simulink model "HighLevelControl2"  (R2020a)
settings: Solver=FixedStepAuto  StartTime=0.0  StopTime=10  FixedStep=0.01  RelTol=1e-3
libraries: fuzblock x1
settings Model: Creator=Sarah Bassem  LastModifiedBy=ElMousel
settings SolverCC: ZeroCrossControl=DisableAll
settings DataIOCC: ReturnWorkspaceOutputs=off
settings DebuggingCC: ArithmeticOperatorsInVariantConditions=warning
settings SFSimCC: SimUseLocalCustomCode=off  CustomCodeUndefinedFunction=UseInterfaceOnly
settings RTWCC: RTWUseLocalCustomCode=off

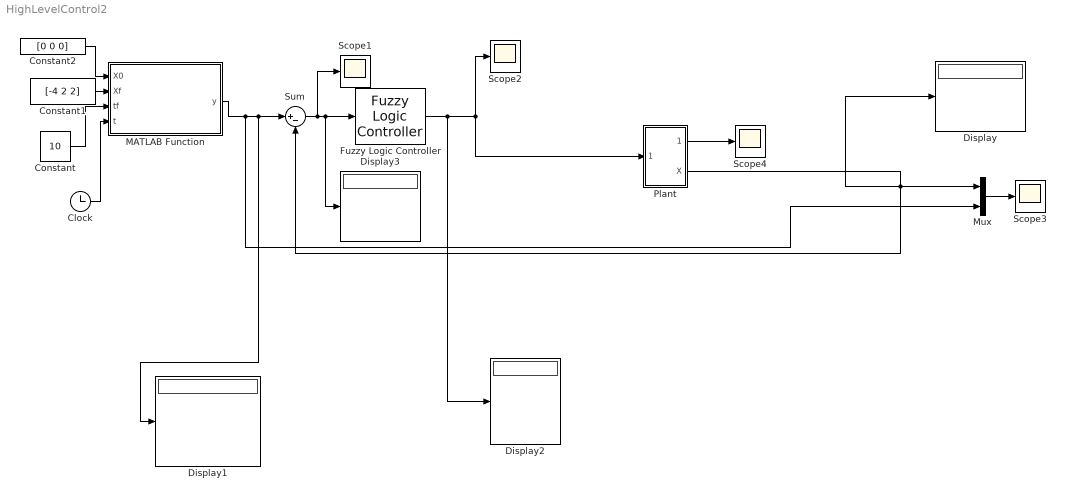
== system HighLevelControl2 ==
  Clock : Clock
  Constant : Constant  Value=10
  Constant1 : Constant  Value=[-4 2 2]
  Constant2 : Constant  Value=[0 0 0]
  Display{,1..3} (4 alike) : Display
  Fuzzy Logic Controller : fuzblock/Fuzzy Logic  Controller  FIS='fuzzyy.fis'  OutputSampleNumber=101  DataType=double  FuzzifiedInputs=off  RuleFiringStrengths=off  RuleOutputs=off  AggregatedOutputs=off  SimulateUsing=Interpreted execution  OutOfRangeInputValueMessage=warning  NoRuleFiredMessage=warning  EmptyOutputFuzzySetMessage=warning
  MATLAB Function : MATLAB Function  TreatAsAtomicUnit=on
  Mux : Mux  Inputs=2
  Plant : Subsystem
  Scope{1..4} (4 alike) : Scope
  Sum : Sum  Inputs=|+-
  wires:
  Sum/1 -> Scope1/1, Display3/1, Fuzzy Logic Controller/1
  MATLAB Function/1(y) -> Mux/2, Display1/1, Sum/1
  Fuzzy Logic Controller/1 -> Display2/1, Plant/1(X_dot), Scope2/1
  Constant/1 -> MATLAB Function/3(tf)
  Constant2/1 -> MATLAB Function/1(X0)
  Clock/1 -> MATLAB Function/4(t)
  Mux/1 -> Scope3/1
  Constant1/1 -> MATLAB Function/2(Xf)
  Plant/2(X) -> Display/1, Mux/1, Sum/2
  Plant/1(q_dot) -> Scope4/1

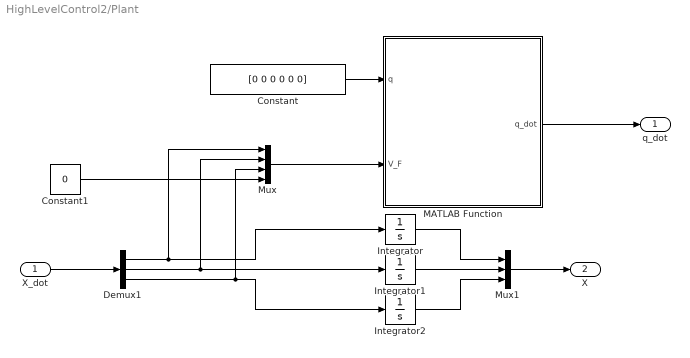
== system HighLevelControl2/Plant ==
  X_dot : Inport
  Constant : Constant  Value=[0 0 0 0 0 0]
  Constant1 : Constant  Value=0
  Demux1 : Demux  Outputs=3
  Integrator : Integrator
  Integrator1 : Integrator
  Integrator2 : Integrator
  MATLAB Function : MATLAB Function  TreatAsAtomicUnit=on
  Mux : Mux
  Mux1 : Mux  Inputs=3
  q_dot : Outport
  X : Outport  Port=2
  wires:
  X_dot/1 -> Demux1/1
  Demux1/1 -> Mux/1, Integrator/1
  Demux1/2 -> Mux/2, Integrator1/1
  Demux1/3 -> Mux/3, Integrator2/1
  Constant/1 -> MATLAB Function/1(q)
  Constant1/1 -> Mux/4
  Mux/1 -> MATLAB Function/2(V_F)
  MATLAB Function/1(q_dot) -> q_dot/1
  Mux1/1 -> X/1
  Integrator/1 -> Mux1/1
  Integrator1/1 -> Mux1/2
  Integrator2/1 -> Mux1/3

== matlab function HighLevelControl2/Plant/MATLAB Function ==
  data: q input; q_dot output; V_F input
function q_dot=inverse_velocity_model(q,V_F)
%j_inv= inverse_jacobian_matrix(q)
 J=jacobian_matrix_num(q);
 r=rank(J)
 b=zeros(4,6);
 q_dot=zeros(6,1);
 for i=1:4
     for j =1:6
         b(i,j)=J(i,j);
     end
 end
 a=b
 r=rank(a)       
%  [RB,p]= rref(J);

j_inv=pinv(b);
x=V_F;
 q_dot=j_inv*V_F

end

== matlab function HighLevelControl2/MATLAB Function ==
  data: X0 input; y output; Xf input; tf input; t input
function y = Ref(X0, Xf, tf,t)
% coder.extrinsic('task_traj_01_first_three_joints');
% y=zeros(3,1);
% y=task_traj_01_first_three_joints(X0, Xf, tf,t);
y = (Xf-X0)*t/tf+(X0);
end
